simulink model "cn_i_128w_2k_do_al_r302"  (Simulink 6.2)
settings: Solver=ode45  StartTime=0.0  StopTime=1000  RelTol=1e-3
libraries: xbsIndex_r3 x481, xps_library x27, ddc_library x4, reorder_library x3, fft_library x2, pfb_library x2, simulink x1, adcscope_lib x1, delay_lib x1
(part 2 of 4)

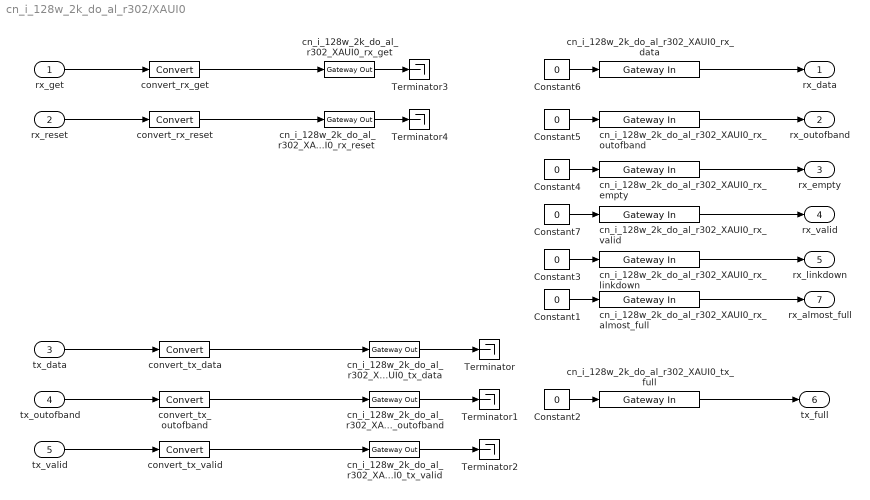
== system cn_i_128w_2k_do_al_r302/XAUI0 ==
  rx_get : Inport  Port=1  LatchInput=off
  rx_reset : Inport  Port=2  LatchInput=off
  tx_data : Inport  Port=3  LatchInput=off
  tx_outofband : Inport  Port=4  LatchInput=off
  tx_valid : Inport  Port=5  LatchInput=off
  Constant{1..7} (7 alike) : Constant  Value=0
  Terminator{,1..4} (5 alike) : Terminator
  cn_i_128w_2k_do_al_r302_XAUI0_rx_almost_full : xbsIndex_r3/Gateway In  arith_type=Boolean  n_bits=1  bin_pt=0  quantization=Truncate  overflow=Wrap  period=1  timing_constraint=None  locs_specified=off  LOCs={}  needs_fixed_name=off  dbl_ovrd=off  show_param=off
      settings: xl_area=[0, 0, 0, 0, 0, 0, 0]
  cn_i_128w_2k_do_al_r302_XAUI0_rx_data : xbsIndex_r3/Gateway In  arith_type=Unsigned  n_bits=64  bin_pt=0  quantization=Truncate  overflow=Wrap  period=1  timing_constraint=None  locs_specified=off  LOCs={}  needs_fixed_name=off  dbl_ovrd=off  show_param=off
      settings: xl_area=[0, 0, 0, 0, 0, 0, 0]
  cn_i_128w_2k_do_al_r302_XAUI0_rx_empty : xbsIndex_r3/Gateway In  arith_type=Boolean  n_bits=1  bin_pt=0  quantization=Truncate  overflow=Wrap  period=1  timing_constraint=None  locs_specified=off  LOCs={}  needs_fixed_name=off  dbl_ovrd=off  show_param=off
      settings: xl_area=[0, 0, 0, 0, 0, 0, 0]
  cn_i_128w_2k_do_al_r302_XAUI0_rx_get : xbsIndex_r3/Gateway Out  output_type=Double  nbits=8  bin_pt=6  arith_type=Boolean  quantization=Truncate  overflow=Wrap  hdl_port=on  timing_constraint=None  locs_specified=off  LOCs={}  needs_fixed_name=off  show_param=off
      settings: xl_area=[0, 0, 0, 0, 0, 0, 0]
  cn_i_128w_2k_do_al_r302_XAUI0_rx_linkdown : xbsIndex_r3/Gateway In  arith_type=Boolean  n_bits=1  bin_pt=0  quantization=Truncate  overflow=Wrap  period=1  timing_constraint=None  locs_specified=off  LOCs={}  needs_fixed_name=off  dbl_ovrd=off  show_param=off
      settings: xl_area=[0, 0, 0, 0, 0, 0, 0]
  cn_i_128w_2k_do_al_r302_XAUI0_rx_outofband : xbsIndex_r3/Gateway In  arith_type=Unsigned  n_bits=8  bin_pt=0  quantization=Truncate  overflow=Wrap  period=1  timing_constraint=None  locs_specified=off  LOCs={}  needs_fixed_name=off  dbl_ovrd=off  show_param=off
      settings: xl_area=[0, 0, 0, 0, 0, 0, 0]
  cn_i_128w_2k_do_al_r302_XAUI0_rx_reset : xbsIndex_r3/Gateway Out  output_type=Double  nbits=8  bin_pt=6  arith_type=Boolean  quantization=Truncate  overflow=Wrap  hdl_port=on  timing_constraint=None  locs_specified=off  LOCs={}  needs_fixed_name=off  show_param=off
      settings: xl_area=[0, 0, 0, 0, 0, 0, 0]
  cn_i_128w_2k_do_al_r302_XAUI0_rx_valid : xbsIndex_r3/Gateway In  arith_type=Boolean  n_bits=1  bin_pt=0  quantization=Truncate  overflow=Wrap  period=1  timing_constraint=None  locs_specified=off  LOCs={}  needs_fixed_name=off  dbl_ovrd=off  show_param=off
      settings: xl_area=[0, 0, 0, 0, 0, 0, 0]
  cn_i_128w_2k_do_al_r302_XAUI0_tx_data : xbsIndex_r3/Gateway Out  output_type=Double  nbits=8  bin_pt=6  arith_type=Boolean  quantization=Truncate  overflow=Wrap  hdl_port=on  timing_constraint=None  locs_specified=off  LOCs={}  needs_fixed_name=off  show_param=off
      settings: xl_area=[0, 0, 0, 0, 0, 0, 0]
  cn_i_128w_2k_do_al_r302_XAUI0_tx_full : xbsIndex_r3/Gateway In  arith_type=Boolean  n_bits=1  bin_pt=0  quantization=Truncate  overflow=Wrap  period=1  timing_constraint=None  locs_specified=off  LOCs={}  needs_fixed_name=off  dbl_ovrd=off  show_param=off
      settings: xl_area=[0, 0, 0, 0, 0, 0, 0]
  cn_i_128w_2k_do_al_r302_XAUI0_tx_outofband : xbsIndex_r3/Gateway Out  output_type=Double  nbits=8  bin_pt=6  arith_type=Boolean  quantization=Truncate  overflow=Wrap  hdl_port=on  timing_constraint=None  locs_specified=off  LOCs={}  needs_fixed_name=off  show_param=off
      settings: xl_area=[0, 0, 0, 0, 0, 0, 0]
  cn_i_128w_2k_do_al_r302_XAUI0_tx_valid : xbsIndex_r3/Gateway Out  output_type=Double  nbits=8  bin_pt=6  arith_type=Boolean  quantization=Truncate  overflow=Wrap  hdl_port=on  timing_constraint=None  locs_specified=off  LOCs={}  needs_fixed_name=off  show_param=off
      settings: xl_area=[0, 0, 0, 0, 0, 0, 0]
  convert_rx_get : xbsIndex_r3/Convert  arith_type=Boolean  n_bits=64  bin_pt=0  quantization=Truncate  overflow=Wrap  latency=0  explicit_period=off  period=1  dbl_ovrd=off  show_param=off  inserted_by_tool=off  pipeline=off
      settings: xl_area=[0, 0, 0, 0, 0, 0, 0]
  convert_rx_reset : xbsIndex_r3/Convert  arith_type=Boolean  n_bits=1  bin_pt=0  quantization=Truncate  overflow=Wrap  latency=0  explicit_period=off  period=1  dbl_ovrd=off  show_param=off  inserted_by_tool=off  pipeline=off
      settings: xl_area=[0, 0, 0, 0, 0, 0, 0]
  convert_tx_data : xbsIndex_r3/Convert  arith_type=Unsigned  n_bits=64  bin_pt=0  quantization=Truncate  overflow=Wrap  latency=0  explicit_period=off  period=1  dbl_ovrd=off  show_param=off  inserted_by_tool=off  pipeline=off
      settings: xl_area=[0, 0, 0, 0, 0, 0, 0]
  convert_tx_outofband : xbsIndex_r3/Convert  arith_type=Unsigned  n_bits=8  bin_pt=0  quantization=Truncate  overflow=Wrap  latency=0  explicit_period=off  period=1  dbl_ovrd=off  show_param=off  inserted_by_tool=off  pipeline=off
      settings: xl_area=[0, 0, 0, 0, 0, 0, 0]
  convert_tx_valid : xbsIndex_r3/Convert  arith_type=Boolean  n_bits=1  bin_pt=0  quantization=Truncate  overflow=Wrap  latency=0  explicit_period=off  period=1  dbl_ovrd=off  show_param=off  inserted_by_tool=off  pipeline=off
      settings: xl_area=[0, 0, 0, 0, 0, 0, 0]
  rx_data : Outport
  rx_outofband : Outport  Port=2
  rx_empty : Outport  Port=3
  rx_valid : Outport  Port=4
  rx_linkdown : Outport  Port=5
  tx_full : Outport  Port=6
  rx_almost_full : Outport  Port=7
  wires:
  Constant1/1 -> cn_i_128w_2k_do_al_r302_XAUI0_rx_almost_full/1
  cn_i_128w_2k_do_al_r302_XAUI0_rx_almost_full/1 -> rx_almost_full/1
  cn_i_128w_2k_do_al_r302_XAUI0_rx_valid/1 -> rx_valid/1
  Constant7/1 -> cn_i_128w_2k_do_al_r302_XAUI0_rx_valid/1
  cn_i_128w_2k_do_al_r302_XAUI0_rx_reset/1 -> Terminator4/1
  cn_i_128w_2k_do_al_r302_XAUI0_rx_get/1 -> Terminator3/1
  Constant6/1 -> cn_i_128w_2k_do_al_r302_XAUI0_rx_data/1
  Constant5/1 -> cn_i_128w_2k_do_al_r302_XAUI0_rx_outofband/1
  Constant4/1 -> cn_i_128w_2k_do_al_r302_XAUI0_rx_empty/1
  Constant3/1 -> cn_i_128w_2k_do_al_r302_XAUI0_rx_linkdown/1
  Constant2/1 -> cn_i_128w_2k_do_al_r302_XAUI0_tx_full/1
  cn_i_128w_2k_do_al_r302_XAUI0_tx_valid/1 -> Terminator2/1
  cn_i_128w_2k_do_al_r302_XAUI0_tx_outofband/1 -> Terminator1/1
  cn_i_128w_2k_do_al_r302_XAUI0_tx_data/1 -> Terminator/1
  cn_i_128w_2k_do_al_r302_XAUI0_tx_full/1 -> tx_full/1
  convert_tx_valid/1 -> cn_i_128w_2k_do_al_r302_XAUI0_tx_valid/1
  tx_valid/1 -> convert_tx_valid/1
  convert_tx_outofband/1 -> cn_i_128w_2k_do_al_r302_XAUI0_tx_outofband/1
  tx_outofband/1 -> convert_tx_outofband/1
  convert_tx_data/1 -> cn_i_128w_2k_do_al_r302_XAUI0_tx_data/1
  tx_data/1 -> convert_tx_data/1
  cn_i_128w_2k_do_al_r302_XAUI0_rx_linkdown/1 -> rx_linkdown/1
  cn_i_128w_2k_do_al_r302_XAUI0_rx_empty/1 -> rx_empty/1
  cn_i_128w_2k_do_al_r302_XAUI0_rx_outofband/1 -> rx_outofband/1
  cn_i_128w_2k_do_al_r302_XAUI0_rx_data/1 -> rx_data/1
  convert_rx_reset/1 -> cn_i_128w_2k_do_al_r302_XAUI0_rx_reset/1
  rx_reset/1 -> convert_rx_reset/1
  convert_rx_get/1 -> cn_i_128w_2k_do_al_r302_XAUI0_rx_get/1
  rx_get/1 -> convert_rx_get/1

== system cn_i_128w_2k_do_al_r302/calc_adc_sum_sq1 ==
  pol_in : Inport  Port=1  LatchInput=off
  accum_rst : Inport  Port=2  LatchInput=off
  Accumulator : xbsIndex_r3/Accumulator  n_bits=32  overflow=Wrap  operation=Add  scale=1  explicit_period=off  period=1  rst=on  hasbypass=off  en=off  dbl_ovrd=off  show_param=off  gen_core=off  use_rpm=on
      settings: xl_area=[0, 0, 0, 0, 0, 0, 0]
  Counter : xbsIndex_r3/Counter  cnt_type=Free Running  n_bits=2  bin_pt=0  arith_type=Unsigned  start_count=0  cnt_to=Inf  cnt_by_val=1  operation=Up  explicit_period=off  period=1  load_pin=off  rst=off  en=off  dbl_ovrd=off  show_param=off  use_rpm=on  gen_core=off
      settings: xl_area=[0, 0, 0, 0, 0, 0, 0]
  Mult : xbsIndex_r3/Mult  precision=Full  arith_type="Signed  (2's comp)"  n_bits=8  bin_pt=2  quantization=Truncate  overflow=Wrap  latency=2  explicit_period=on  period=1  en=off  dbl_ovrd=off  show_param=off  mult_type=Parallel  oversample=2  use_embedded=off  pipeline=on  use_rpm=on  placement_style=Rectangular Shape  gen_core=off
      settings: xl_area=[0, 0, 0, 0, 0, 0, 0]
  Mux : xbsIndex_r3/Mux  inputs=4  precision=Full  arith_type="Signed  (2's comp)"  n_bits=8  bin_pt=2  quantization=Truncate  overflow=Wrap  latency=1  explicit_period=off  period=1  en=off  dbl_ovrd=off  show_param=off  mux_type=off  use_rpm=off  gen_core=off
      settings: xl_area=[0, 0, 0, 0, 0, 0, 0]
  Register : xbsIndex_r3/Register  init=0  reg_only_valid=off  explicit_period=off  period=1  rst=off  en=on  out_en=off  dbl_ovrd=off  show_param=off
      settings: xl_area=[0, 0, 0, 0, 0, 0, 0]
  decat4 : Subsystem
  sum_sq : Outport
  wires:
  Mult/1 -> Accumulator/1
  Accumulator/1 -> Register/1
  Register/1 -> sum_sq/1
  Mux/1 -> Mult/1, Mult/2
  Counter/1 -> Mux/1
  accum_rst/1 -> Accumulator/2, Register/2
  pol_in/1 -> decat4/1(In1)
  decat4/1(Out1) -> Mux/2
  decat4/2(Out2) -> Mux/4
  decat4/3(Out3) -> Mux/3
  decat4/4(Out4) -> Mux/5

== system cn_i_128w_2k_do_al_r302/calc_adc_sum_sq2 ==
  pol_in : Inport  Port=1  LatchInput=off
  accum_rst : Inport  Port=2  LatchInput=off
  Accumulator : xbsIndex_r3/Accumulator  n_bits=32  overflow=Wrap  operation=Add  scale=1  explicit_period=off  period=1  rst=on  hasbypass=off  en=off  dbl_ovrd=off  show_param=off  gen_core=off  use_rpm=on
      settings: xl_area=[0, 0, 0, 0, 0, 0, 0]
  Counter : xbsIndex_r3/Counter  cnt_type=Free Running  n_bits=2  bin_pt=0  arith_type=Unsigned  start_count=0  cnt_to=Inf  cnt_by_val=1  operation=Up  explicit_period=off  period=1  load_pin=off  rst=off  en=off  dbl_ovrd=off  show_param=off  use_rpm=on  gen_core=off
      settings: xl_area=[0, 0, 0, 0, 0, 0, 0]
  Mult : xbsIndex_r3/Mult  precision=Full  arith_type="Signed  (2's comp)"  n_bits=8  bin_pt=2  quantization=Truncate  overflow=Wrap  latency=2  explicit_period=on  period=1  en=off  dbl_ovrd=off  show_param=off  mult_type=Parallel  oversample=2  use_embedded=off  pipeline=on  use_rpm=on  placement_style=Rectangular Shape  gen_core=off
      settings: xl_area=[0, 0, 0, 0, 0, 0, 0]
  Mux : xbsIndex_r3/Mux  inputs=4  precision=Full  arith_type="Signed  (2's comp)"  n_bits=8  bin_pt=2  quantization=Truncate  overflow=Wrap  latency=1  explicit_period=off  period=1  en=off  dbl_ovrd=off  show_param=off  mux_type=off  use_rpm=off  gen_core=off
      settings: xl_area=[0, 0, 0, 0, 0, 0, 0]
  Register : xbsIndex_r3/Register  init=0  reg_only_valid=off  explicit_period=off  period=1  rst=off  en=on  out_en=off  dbl_ovrd=off  show_param=off
      settings: xl_area=[0, 0, 0, 0, 0, 0, 0]
  decat4 : Subsystem
  sum_sq : Outport
  wires:
  Mult/1 -> Accumulator/1
  Accumulator/1 -> Register/1
  Register/1 -> sum_sq/1
  Mux/1 -> Mult/1, Mult/2
  Counter/1 -> Mux/1
  accum_rst/1 -> Accumulator/2, Register/2
  pol_in/1 -> decat4/1(In1)
  decat4/1(Out1) -> Mux/2
  decat4/2(Out2) -> Mux/4
  decat4/3(Out3) -> Mux/3
  decat4/4(Out4) -> Mux/5

== system cn_i_128w_2k_do_al_r302/calc_adc_sum_sq3 ==
  pol_in : Inport  Port=1  LatchInput=off
  accum_rst : Inport  Port=2  LatchInput=off
  Accumulator : xbsIndex_r3/Accumulator  n_bits=32  overflow=Wrap  operation=Add  scale=1  explicit_period=off  period=1  rst=on  hasbypass=off  en=off  dbl_ovrd=off  show_param=off  gen_core=off  use_rpm=on
      settings: xl_area=[0, 0, 0, 0, 0, 0, 0]
  Counter : xbsIndex_r3/Counter  cnt_type=Free Running  n_bits=2  bin_pt=0  arith_type=Unsigned  start_count=0  cnt_to=Inf  cnt_by_val=1  operation=Up  explicit_period=off  period=1  load_pin=off  rst=off  en=off  dbl_ovrd=off  show_param=off  use_rpm=on  gen_core=off
      settings: xl_area=[0, 0, 0, 0, 0, 0, 0]
  Mult : xbsIndex_r3/Mult  precision=Full  arith_type="Signed  (2's comp)"  n_bits=8  bin_pt=2  quantization=Truncate  overflow=Wrap  latency=2  explicit_period=on  period=1  en=off  dbl_ovrd=off  show_param=off  mult_type=Parallel  oversample=2  use_embedded=off  pipeline=on  use_rpm=on  placement_style=Rectangular Shape  gen_core=off
      settings: xl_area=[0, 0, 0, 0, 0, 0, 0]
  Mux : xbsIndex_r3/Mux  inputs=4  precision=Full  arith_type="Signed  (2's comp)"  n_bits=8  bin_pt=2  quantization=Truncate  overflow=Wrap  latency=1  explicit_period=off  period=1  en=off  dbl_ovrd=off  show_param=off  mux_type=off  use_rpm=off  gen_core=off
      settings: xl_area=[0, 0, 0, 0, 0, 0, 0]
  Register : xbsIndex_r3/Register  init=0  reg_only_valid=off  explicit_period=off  period=1  rst=off  en=on  out_en=off  dbl_ovrd=off  show_param=off
      settings: xl_area=[0, 0, 0, 0, 0, 0, 0]
  decat4 : Subsystem
  sum_sq : Outport
  wires:
  Mult/1 -> Accumulator/1
  Accumulator/1 -> Register/1
  Register/1 -> sum_sq/1
  Mux/1 -> Mult/1, Mult/2
  Counter/1 -> Mux/1
  accum_rst/1 -> Accumulator/2, Register/2
  pol_in/1 -> decat4/1(In1)
  decat4/1(Out1) -> Mux/2
  decat4/2(Out2) -> Mux/4
  decat4/3(Out3) -> Mux/3
  decat4/4(Out4) -> Mux/5

== system cn_i_128w_2k_do_al_r302/calc_adc_sum_sq4 ==
  pol_in : Inport  Port=1  LatchInput=off
  accum_rst : Inport  Port=2  LatchInput=off
  Accumulator : xbsIndex_r3/Accumulator  n_bits=32  overflow=Wrap  operation=Add  scale=1  explicit_period=off  period=1  rst=on  hasbypass=off  en=off  dbl_ovrd=off  show_param=off  gen_core=off  use_rpm=on
      settings: xl_area=[0, 0, 0, 0, 0, 0, 0]
  Counter : xbsIndex_r3/Counter  cnt_type=Free Running  n_bits=2  bin_pt=0  arith_type=Unsigned  start_count=0  cnt_to=Inf  cnt_by_val=1  operation=Up  explicit_period=off  period=1  load_pin=off  rst=off  en=off  dbl_ovrd=off  show_param=off  use_rpm=on  gen_core=off
      settings: xl_area=[0, 0, 0, 0, 0, 0, 0]
  Mult : xbsIndex_r3/Mult  precision=Full  arith_type="Signed  (2's comp)"  n_bits=8  bin_pt=2  quantization=Truncate  overflow=Wrap  latency=2  explicit_period=on  period=1  en=off  dbl_ovrd=off  show_param=off  mult_type=Parallel  oversample=2  use_embedded=off  pipeline=on  use_rpm=on  placement_style=Rectangular Shape  gen_core=off
      settings: xl_area=[0, 0, 0, 0, 0, 0, 0]
  Mux : xbsIndex_r3/Mux  inputs=4  precision=Full  arith_type="Signed  (2's comp)"  n_bits=8  bin_pt=2  quantization=Truncate  overflow=Wrap  latency=1  explicit_period=off  period=1  en=off  dbl_ovrd=off  show_param=off  mux_type=off  use_rpm=off  gen_core=off
      settings: xl_area=[0, 0, 0, 0, 0, 0, 0]
  Register : xbsIndex_r3/Register  init=0  reg_only_valid=off  explicit_period=off  period=1  rst=off  en=on  out_en=off  dbl_ovrd=off  show_param=off
      settings: xl_area=[0, 0, 0, 0, 0, 0, 0]
  decat4 : Subsystem
  sum_sq : Outport
  wires:
  Mult/1 -> Accumulator/1
  Accumulator/1 -> Register/1
  Register/1 -> sum_sq/1
  Mux/1 -> Mult/1, Mult/2
  Counter/1 -> Mux/1
  accum_rst/1 -> Accumulator/2, Register/2
  pol_in/1 -> decat4/1(In1)
  decat4/1(Out1) -> Mux/2
  decat4/2(Out2) -> Mux/4
  decat4/3(Out3) -> Mux/3
  decat4/4(Out4) -> Mux/5

== system cn_i_128w_2k_do_al_r302/concat ==
  In1 : Inport  Port=1  LatchInput=off
  In2 : Inport  Port=2  LatchInput=off
  In3 : Inport  Port=3  LatchInput=off
  In4 : Inport  Port=4  LatchInput=off
  Concat2 : xbsIndex_r3/Concat  num_inputs=4  explicit_period=off  period=1  dbl_ovrd=off
  R1 : xbsIndex_r3/Reinterpret  force_arith_type=on  arith_type=Unsigned  force_bin_pt=on  bin_pt=0  force_valid=on
  R2 : xbsIndex_r3/Reinterpret  force_arith_type=on  arith_type=Unsigned  force_bin_pt=on  bin_pt=0  force_valid=on
  R3 : xbsIndex_r3/Reinterpret  force_arith_type=on  arith_type=Unsigned  force_bin_pt=on  bin_pt=0  force_valid=on
  Reinterpret2 : xbsIndex_r3/Reinterpret  force_arith_type=on  arith_type=Unsigned  force_bin_pt=on  bin_pt=0  force_valid=on
  Out1 : Outport
  wires:
  Reinterpret2/1 -> Concat2/1
  R1/1 -> Concat2/2
  R2/1 -> Concat2/3
  R3/1 -> Concat2/4
  In1/1 -> Reinterpret2/1
  In2/1 -> R1/1
  In3/1 -> R2/1
  In4/1 -> R3/1
  Concat2/1 -> Out1/1

== system cn_i_128w_2k_do_al_r302/concat4 ==
  In1 : Inport  Port=1  LatchInput=off
  In2 : Inport  Port=2  LatchInput=off
  In3 : Inport  Port=3  LatchInput=off
  In4 : Inport  Port=4  LatchInput=off
  Concat2 : xbsIndex_r3/Concat  num_inputs=4  explicit_period=off  period=1  dbl_ovrd=off
  R1 : xbsIndex_r3/Reinterpret  force_arith_type=on  arith_type=Unsigned  force_bin_pt=on  bin_pt=0  force_valid=on
  R2 : xbsIndex_r3/Reinterpret  force_arith_type=on  arith_type=Unsigned  force_bin_pt=on  bin_pt=0  force_valid=on
  R3 : xbsIndex_r3/Reinterpret  force_arith_type=on  arith_type=Unsigned  force_bin_pt=on  bin_pt=0  force_valid=on
  Reinterpret2 : xbsIndex_r3/Reinterpret  force_arith_type=on  arith_type=Unsigned  force_bin_pt=on  bin_pt=0  force_valid=on
  Out1 : Outport
  wires:
  Concat2/1 -> Out1/1
  In4/1 -> R3/1
  In3/1 -> R2/1
  In2/1 -> R1/1
  In1/1 -> Reinterpret2/1
  R3/1 -> Concat2/4
  R2/1 -> Concat2/3
  R1/1 -> Concat2/2
  Reinterpret2/1 -> Concat2/1

== system cn_i_128w_2k_do_al_r302/concat5 ==
  In1 : Inport  Port=1  LatchInput=off
  In2 : Inport  Port=2  LatchInput=off
  In3 : Inport  Port=3  LatchInput=off
  In4 : Inport  Port=4  LatchInput=off
  Concat2 : xbsIndex_r3/Concat  num_inputs=4  explicit_period=off  period=1  dbl_ovrd=off
  R1 : xbsIndex_r3/Reinterpret  force_arith_type=on  arith_type=Unsigned  force_bin_pt=on  bin_pt=0  force_valid=on
  R2 : xbsIndex_r3/Reinterpret  force_arith_type=on  arith_type=Unsigned  force_bin_pt=on  bin_pt=0  force_valid=on
  R3 : xbsIndex_r3/Reinterpret  force_arith_type=on  arith_type=Unsigned  force_bin_pt=on  bin_pt=0  force_valid=on
  Reinterpret2 : xbsIndex_r3/Reinterpret  force_arith_type=on  arith_type=Unsigned  force_bin_pt=on  bin_pt=0  force_valid=on
  Out1 : Outport
  wires:
  Reinterpret2/1 -> Concat2/1
  R1/1 -> Concat2/2
  R2/1 -> Concat2/3
  R3/1 -> Concat2/4
  In1/1 -> Reinterpret2/1
  In2/1 -> R1/1
  In3/1 -> R2/1
  In4/1 -> R3/1
  Concat2/1 -> Out1/1

== system cn_i_128w_2k_do_al_r302/concat6 ==
  In1 : Inport  Port=1  LatchInput=off
  In2 : Inport  Port=2  LatchInput=off
  In3 : Inport  Port=3  LatchInput=off
  In4 : Inport  Port=4  LatchInput=off
  Concat2 : xbsIndex_r3/Concat  num_inputs=4  explicit_period=off  period=1  dbl_ovrd=off
  R1 : xbsIndex_r3/Reinterpret  force_arith_type=on  arith_type=Unsigned  force_bin_pt=on  bin_pt=0  force_valid=on
  R2 : xbsIndex_r3/Reinterpret  force_arith_type=on  arith_type=Unsigned  force_bin_pt=on  bin_pt=0  force_valid=on
  R3 : xbsIndex_r3/Reinterpret  force_arith_type=on  arith_type=Unsigned  force_bin_pt=on  bin_pt=0  force_valid=on
  Reinterpret2 : xbsIndex_r3/Reinterpret  force_arith_type=on  arith_type=Unsigned  force_bin_pt=on  bin_pt=0  force_valid=on
  Out1 : Outport
  wires:
  Concat2/1 -> Out1/1
  In4/1 -> R3/1
  In3/1 -> R2/1
  In2/1 -> R1/1
  In1/1 -> Reinterpret2/1
  R3/1 -> Concat2/4
  R2/1 -> Concat2/3
  R1/1 -> Concat2/2
  Reinterpret2/1 -> Concat2/1

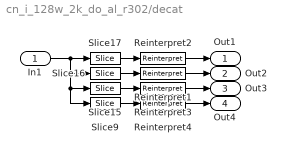
== system cn_i_128w_2k_do_al_r302/decat ==
  In1 : Inport  Port=1  LatchInput=off
  Reinterpret{1..4} (4 alike) : xbsIndex_r3/Reinterpret  force_arith_type=on  arith_type="Signed  (2's comp)"  force_bin_pt=on  bin_pt=7  force_valid=on
  Slice15 : xbsIndex_r3/Slice  mode=Lower Bit Location + Width  nbits=8  bit1=0  base1=MSB of Input  bit0=8  base0=LSB of Input  boolean_output=off  explicit_period=off  period=1  dbl_ovrd=off
  Slice16 : xbsIndex_r3/Slice  mode=Lower Bit Location + Width  nbits=8  bit1=0  base1=MSB of Input  bit0=16  base0=LSB of Input  boolean_output=off  explicit_period=off  period=1  dbl_ovrd=off
  Slice17 : xbsIndex_r3/Slice  mode=Lower Bit Location + Width  nbits=8  bit1=0  base1=MSB of Input  bit0=24  base0=LSB of Input  boolean_output=off  explicit_period=off  period=1  dbl_ovrd=off
  Slice9 : xbsIndex_r3/Slice  mode=Lower Bit Location + Width  nbits=8  bit1=0  base1=MSB of Input  bit0=0  base0=LSB of Input  boolean_output=off  explicit_period=off  period=1  dbl_ovrd=off
  Out1 : Outport
  Out2 : Outport  Port=2
  Out3 : Outport  Port=3
  Out4 : Outport  Port=4
  wires:
  In1/1 -> Slice17/1, Slice16/1, Slice9/1, Slice15/1
  Slice17/1 -> Reinterpret2/1
  Slice16/1 -> Reinterpret1/1
  Slice15/1 -> Reinterpret3/1
  Slice9/1 -> Reinterpret4/1
  Reinterpret2/1 -> Out1/1
  Reinterpret1/1 -> Out2/1
  Reinterpret3/1 -> Out3/1
  Reinterpret4/1 -> Out4/1

== system cn_i_128w_2k_do_al_r302/decat1 ==
  In1 : Inport  Port=1  LatchInput=off
  Reinterpret{1..4} (4 alike) : xbsIndex_r3/Reinterpret  force_arith_type=on  arith_type="Signed  (2's comp)"  force_bin_pt=on  bin_pt=7  force_valid=on
  Slice15 : xbsIndex_r3/Slice  mode=Lower Bit Location + Width  nbits=8  bit1=0  base1=MSB of Input  bit0=8  base0=LSB of Input  boolean_output=off  explicit_period=off  period=1  dbl_ovrd=off
  Slice16 : xbsIndex_r3/Slice  mode=Lower Bit Location + Width  nbits=8  bit1=0  base1=MSB of Input  bit0=16  base0=LSB of Input  boolean_output=off  explicit_period=off  period=1  dbl_ovrd=off
  Slice17 : xbsIndex_r3/Slice  mode=Lower Bit Location + Width  nbits=8  bit1=0  base1=MSB of Input  bit0=24  base0=LSB of Input  boolean_output=off  explicit_period=off  period=1  dbl_ovrd=off
  Slice9 : xbsIndex_r3/Slice  mode=Lower Bit Location + Width  nbits=8  bit1=0  base1=MSB of Input  bit0=0  base0=LSB of Input  boolean_output=off  explicit_period=off  period=1  dbl_ovrd=off
  Out1 : Outport
  Out2 : Outport  Port=2
  Out3 : Outport  Port=3
  Out4 : Outport  Port=4
  wires:
  Reinterpret4/1 -> Out4/1
  Reinterpret3/1 -> Out3/1
  Reinterpret1/1 -> Out2/1
  Reinterpret2/1 -> Out1/1
  Slice9/1 -> Reinterpret4/1
  Slice15/1 -> Reinterpret3/1
  Slice16/1 -> Reinterpret1/1
  Slice17/1 -> Reinterpret2/1
  In1/1 -> Slice15/1, Slice9/1, Slice16/1, Slice17/1

== system cn_i_128w_2k_do_al_r302/decat2 ==
  In1 : Inport  Port=1  LatchInput=off
  Reinterpret{1..4} (4 alike) : xbsIndex_r3/Reinterpret  force_arith_type=on  arith_type="Signed  (2's comp)"  force_bin_pt=on  bin_pt=7  force_valid=on
  Slice15 : xbsIndex_r3/Slice  mode=Lower Bit Location + Width  nbits=8  bit1=0  base1=MSB of Input  bit0=8  base0=LSB of Input  boolean_output=off  explicit_period=off  period=1  dbl_ovrd=off
  Slice16 : xbsIndex_r3/Slice  mode=Lower Bit Location + Width  nbits=8  bit1=0  base1=MSB of Input  bit0=16  base0=LSB of Input  boolean_output=off  explicit_period=off  period=1  dbl_ovrd=off
  Slice17 : xbsIndex_r3/Slice  mode=Lower Bit Location + Width  nbits=8  bit1=0  base1=MSB of Input  bit0=24  base0=LSB of Input  boolean_output=off  explicit_period=off  period=1  dbl_ovrd=off
  Slice9 : xbsIndex_r3/Slice  mode=Lower Bit Location + Width  nbits=8  bit1=0  base1=MSB of Input  bit0=0  base0=LSB of Input  boolean_output=off  explicit_period=off  period=1  dbl_ovrd=off
  Out1 : Outport
  Out2 : Outport  Port=2
  Out3 : Outport  Port=3
  Out4 : Outport  Port=4
  wires:
  Reinterpret4/1 -> Out4/1
  Reinterpret3/1 -> Out3/1
  Reinterpret1/1 -> Out2/1
  Reinterpret2/1 -> Out1/1
  Slice9/1 -> Reinterpret4/1
  Slice15/1 -> Reinterpret3/1
  Slice16/1 -> Reinterpret1/1
  Slice17/1 -> Reinterpret2/1
  In1/1 -> Slice15/1, Slice9/1, Slice16/1, Slice17/1

== system cn_i_128w_2k_do_al_r302/decat3 ==
  In1 : Inport  Port=1  LatchInput=off
  Reinterpret{1..4} (4 alike) : xbsIndex_r3/Reinterpret  force_arith_type=on  arith_type="Signed  (2's comp)"  force_bin_pt=on  bin_pt=7  force_valid=on
  Slice15 : xbsIndex_r3/Slice  mode=Lower Bit Location + Width  nbits=8  bit1=0  base1=MSB of Input  bit0=8  base0=LSB of Input  boolean_output=off  explicit_period=off  period=1  dbl_ovrd=off
  Slice16 : xbsIndex_r3/Slice  mode=Lower Bit Location + Width  nbits=8  bit1=0  base1=MSB of Input  bit0=16  base0=LSB of Input  boolean_output=off  explicit_period=off  period=1  dbl_ovrd=off
  Slice17 : xbsIndex_r3/Slice  mode=Lower Bit Location + Width  nbits=8  bit1=0  base1=MSB of Input  bit0=24  base0=LSB of Input  boolean_output=off  explicit_period=off  period=1  dbl_ovrd=off
  Slice9 : xbsIndex_r3/Slice  mode=Lower Bit Location + Width  nbits=8  bit1=0  base1=MSB of Input  bit0=0  base0=LSB of Input  boolean_output=off  explicit_period=off  period=1  dbl_ovrd=off
  Out1 : Outport
  Out2 : Outport  Port=2
  Out3 : Outport  Port=3
  Out4 : Outport  Port=4
  wires:
  In1/1 -> Slice17/1, Slice16/1, Slice9/1, Slice15/1
  Slice17/1 -> Reinterpret2/1
  Slice16/1 -> Reinterpret1/1
  Slice15/1 -> Reinterpret3/1
  Slice9/1 -> Reinterpret4/1
  Reinterpret2/1 -> Out1/1
  Reinterpret1/1 -> Out2/1
  Reinterpret3/1 -> Out3/1
  Reinterpret4/1 -> Out4/1

== system cn_i_128w_2k_do_al_r302/downshift ==
  din : Inport  Port=1  LatchInput=off
  Concat : xbsIndex_r3/Concat  num_inputs=2  explicit_period=off  period=1  dbl_ovrd=off
  Convert1 : xbsIndex_r3/Convert  arith_type="Signed  (2's comp)"  n_bits=18  bin_pt=15  quantization="Round  (unbiased: Even Values)"  overflow=Wrap  latency=2  explicit_period=off  period=1  dbl_ovrd=off  show_param=off  inserted_by_tool=off  pipeline=off
      settings: xl_area=[0, 0, 0, 0, 0, 0, 0]
  Convert2 : xbsIndex_r3/Convert  arith_type="Signed  (2's comp)"  n_bits=18  bin_pt=15  quantization="Round  (unbiased: Even Values)"  overflow=Wrap  latency=2  explicit_period=off  period=1  dbl_ovrd=off  show_param=off  inserted_by_tool=off  pipeline=off
      settings: xl_area=[0, 0, 0, 0, 0, 0, 0]
  Reinterpret : xbsIndex_r3/Reinterpret  force_arith_type=on  arith_type="Signed  (2's comp)"  force_bin_pt=on  bin_pt=17  force_valid=on
  Reinterpret1 : xbsIndex_r3/Reinterpret  force_arith_type=on  arith_type="Signed  (2's comp)"  force_bin_pt=on  bin_pt=17  force_valid=on
  Reinterpret3 : xbsIndex_r3/Reinterpret  force_arith_type=on  arith_type=Unsigned  force_bin_pt=on  bin_pt=0  force_valid=on
  Reinterpret4 : xbsIndex_r3/Reinterpret  force_arith_type=on  arith_type=Unsigned  force_bin_pt=on  bin_pt=0  force_valid=on
  Slice2 : xbsIndex_r3/Slice  mode=Upper Bit Location + Width  nbits=18  bit1=0  base1=MSB of Input  bit0=0  base0=LSB of Input  boolean_output=off  explicit_period=off  period=1  dbl_ovrd=off
  Slice20 : xbsIndex_r3/Slice  mode=Lower Bit Location + Width  nbits=18  bit1=0  base1=MSB of Input  bit0=0  base0=LSB of Input  boolean_output=off  explicit_period=off  period=1  dbl_ovrd=off
  dout : Outport
  wires:
  Slice2/1 -> Reinterpret/1
  Slice20/1 -> Reinterpret1/1
  din/1 -> Slice2/1, Slice20/1
  Reinterpret3/1 -> Concat/1
  Reinterpret4/1 -> Concat/2
  Concat/1 -> dout/1
  Reinterpret/1 -> Convert2/1
  Reinterpret1/1 -> Convert1/1
  Convert2/1 -> Reinterpret3/1
  Convert1/1 -> Reinterpret4/1

== system cn_i_128w_2k_do_al_r302/downshift1 ==
  din : Inport  Port=1  LatchInput=off
  Concat : xbsIndex_r3/Concat  num_inputs=2  explicit_period=off  period=1  dbl_ovrd=off
  Convert1 : xbsIndex_r3/Convert  arith_type="Signed  (2's comp)"  n_bits=18  bin_pt=15  quantization="Round  (unbiased: Even Values)"  overflow=Wrap  latency=2  explicit_period=off  period=1  dbl_ovrd=off  show_param=off  inserted_by_tool=off  pipeline=off
      settings: xl_area=[0, 0, 0, 0, 0, 0, 0]
  Convert2 : xbsIndex_r3/Convert  arith_type="Signed  (2's comp)"  n_bits=18  bin_pt=15  quantization="Round  (unbiased: Even Values)"  overflow=Wrap  latency=2  explicit_period=off  period=1  dbl_ovrd=off  show_param=off  inserted_by_tool=off  pipeline=off
      settings: xl_area=[0, 0, 0, 0, 0, 0, 0]
  Reinterpret : xbsIndex_r3/Reinterpret  force_arith_type=on  arith_type="Signed  (2's comp)"  force_bin_pt=on  bin_pt=17  force_valid=on
  Reinterpret1 : xbsIndex_r3/Reinterpret  force_arith_type=on  arith_type="Signed  (2's comp)"  force_bin_pt=on  bin_pt=17  force_valid=on
  Reinterpret3 : xbsIndex_r3/Reinterpret  force_arith_type=on  arith_type=Unsigned  force_bin_pt=on  bin_pt=0  force_valid=on
  Reinterpret4 : xbsIndex_r3/Reinterpret  force_arith_type=on  arith_type=Unsigned  force_bin_pt=on  bin_pt=0  force_valid=on
  Slice2 : xbsIndex_r3/Slice  mode=Upper Bit Location + Width  nbits=18  bit1=0  base1=MSB of Input  bit0=0  base0=LSB of Input  boolean_output=off  explicit_period=off  period=1  dbl_ovrd=off
  Slice20 : xbsIndex_r3/Slice  mode=Lower Bit Location + Width  nbits=18  bit1=0  base1=MSB of Input  bit0=0  base0=LSB of Input  boolean_output=off  explicit_period=off  period=1  dbl_ovrd=off
  dout : Outport
  wires:
  Convert1/1 -> Reinterpret4/1
  Convert2/1 -> Reinterpret3/1
  Reinterpret1/1 -> Convert1/1
  Reinterpret/1 -> Convert2/1
  Concat/1 -> dout/1
  Reinterpret4/1 -> Concat/2
  Reinterpret3/1 -> Concat/1
  din/1 -> Slice20/1, Slice2/1
  Slice20/1 -> Reinterpret1/1
  Slice2/1 -> Reinterpret/1

== system cn_i_128w_2k_do_al_r302/downshift2 ==
  din : Inport  Port=1  LatchInput=off
  Concat : xbsIndex_r3/Concat  num_inputs=2  explicit_period=off  period=1  dbl_ovrd=off
  Convert1 : xbsIndex_r3/Convert  arith_type="Signed  (2's comp)"  n_bits=18  bin_pt=15  quantization="Round  (unbiased: Even Values)"  overflow=Wrap  latency=2  explicit_period=off  period=1  dbl_ovrd=off  show_param=off  inserted_by_tool=off  pipeline=off
      settings: xl_area=[0, 0, 0, 0, 0, 0, 0]
  Convert2 : xbsIndex_r3/Convert  arith_type="Signed  (2's comp)"  n_bits=18  bin_pt=15  quantization="Round  (unbiased: Even Values)"  overflow=Wrap  latency=2  explicit_period=off  period=1  dbl_ovrd=off  show_param=off  inserted_by_tool=off  pipeline=off
      settings: xl_area=[0, 0, 0, 0, 0, 0, 0]
  Reinterpret : xbsIndex_r3/Reinterpret  force_arith_type=on  arith_type="Signed  (2's comp)"  force_bin_pt=on  bin_pt=17  force_valid=on
  Reinterpret1 : xbsIndex_r3/Reinterpret  force_arith_type=on  arith_type="Signed  (2's comp)"  force_bin_pt=on  bin_pt=17  force_valid=on
  Reinterpret3 : xbsIndex_r3/Reinterpret  force_arith_type=on  arith_type=Unsigned  force_bin_pt=on  bin_pt=0  force_valid=on
  Reinterpret4 : xbsIndex_r3/Reinterpret  force_arith_type=on  arith_type=Unsigned  force_bin_pt=on  bin_pt=0  force_valid=on
  Slice2 : xbsIndex_r3/Slice  mode=Upper Bit Location + Width  nbits=18  bit1=0  base1=MSB of Input  bit0=0  base0=LSB of Input  boolean_output=off  explicit_period=off  period=1  dbl_ovrd=off
  Slice20 : xbsIndex_r3/Slice  mode=Lower Bit Location + Width  nbits=18  bit1=0  base1=MSB of Input  bit0=0  base0=LSB of Input  boolean_output=off  explicit_period=off  period=1  dbl_ovrd=off
  dout : Outport
  wires:
  Convert1/1 -> Reinterpret4/1
  Convert2/1 -> Reinterpret3/1
  Reinterpret1/1 -> Convert1/1
  Reinterpret/1 -> Convert2/1
  Concat/1 -> dout/1
  Reinterpret4/1 -> Concat/2
  Reinterpret3/1 -> Concat/1
  din/1 -> Slice20/1, Slice2/1
  Slice20/1 -> Reinterpret1/1
  Slice2/1 -> Reinterpret/1

== system cn_i_128w_2k_do_al_r302/downshift3 ==
  din : Inport  Port=1  LatchInput=off
  Concat : xbsIndex_r3/Concat  num_inputs=2  explicit_period=off  period=1  dbl_ovrd=off
  Convert1 : xbsIndex_r3/Convert  arith_type="Signed  (2's comp)"  n_bits=18  bin_pt=15  quantization="Round  (unbiased: Even Values)"  overflow=Wrap  latency=2  explicit_period=off  period=1  dbl_ovrd=off  show_param=off  inserted_by_tool=off  pipeline=off
      settings: xl_area=[0, 0, 0, 0, 0, 0, 0]
  Convert2 : xbsIndex_r3/Convert  arith_type="Signed  (2's comp)"  n_bits=18  bin_pt=15  quantization="Round  (unbiased: Even Values)"  overflow=Wrap  latency=2  explicit_period=off  period=1  dbl_ovrd=off  show_param=off  inserted_by_tool=off  pipeline=off
      settings: xl_area=[0, 0, 0, 0, 0, 0, 0]
  Reinterpret : xbsIndex_r3/Reinterpret  force_arith_type=on  arith_type="Signed  (2's comp)"  force_bin_pt=on  bin_pt=17  force_valid=on
  Reinterpret1 : xbsIndex_r3/Reinterpret  force_arith_type=on  arith_type="Signed  (2's comp)"  force_bin_pt=on  bin_pt=17  force_valid=on
  Reinterpret3 : xbsIndex_r3/Reinterpret  force_arith_type=on  arith_type=Unsigned  force_bin_pt=on  bin_pt=0  force_valid=on
  Reinterpret4 : xbsIndex_r3/Reinterpret  force_arith_type=on  arith_type=Unsigned  force_bin_pt=on  bin_pt=0  force_valid=on
  Slice2 : xbsIndex_r3/Slice  mode=Upper Bit Location + Width  nbits=18  bit1=0  base1=MSB of Input  bit0=0  base0=LSB of Input  boolean_output=off  explicit_period=off  period=1  dbl_ovrd=off
  Slice20 : xbsIndex_r3/Slice  mode=Lower Bit Location + Width  nbits=18  bit1=0  base1=MSB of Input  bit0=0  base0=LSB of Input  boolean_output=off  explicit_period=off  period=1  dbl_ovrd=off
  dout : Outport
  wires:
  Slice2/1 -> Reinterpret/1
  Slice20/1 -> Reinterpret1/1
  din/1 -> Slice2/1, Slice20/1
  Reinterpret3/1 -> Concat/1
  Reinterpret4/1 -> Concat/2
  Concat/1 -> dout/1
  Reinterpret/1 -> Convert2/1
  Reinterpret1/1 -> Convert1/1
  Convert2/1 -> Reinterpret3/1
  Convert1/1 -> Reinterpret4/1

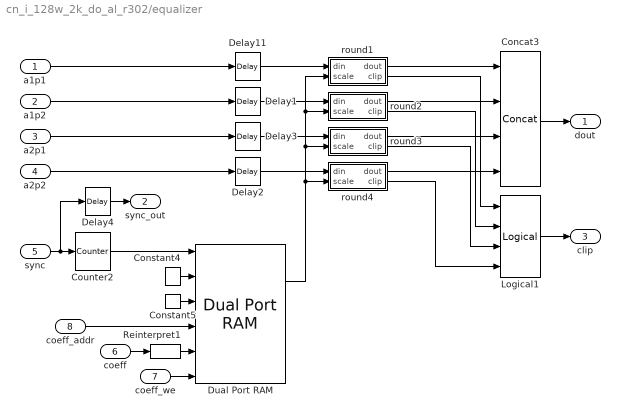
== system cn_i_128w_2k_do_al_r302/equalizer ==
  a1p1 : Inport  Port=1  LatchInput=off
  a1p2 : Inport  Port=2  LatchInput=off
  a2p1 : Inport  Port=3  LatchInput=off
  a2p2 : Inport  Port=4  LatchInput=off
  sync : Inport  Port=5  LatchInput=off
  coeff : Inport  Port=6  LatchInput=off
  coeff_we : Inport  Port=7  LatchInput=off
  coeff_addr : Inport  Port=8  LatchInput=off
  Concat3 : xbsIndex_r3/Concat  num_inputs=4  explicit_period=off  period=1  dbl_ovrd=off
  Constant4 : xbsIndex_r3/Constant  const=0  equ=P=C  arith_type=Unsigned  n_bits=17  bin_pt=3  opselect=C  inp2=PCIN>>17  opr=+  inp1=P  carry=CIN  iostate=0  explicit_period=on  period=1  dbl_ovrd=off
  Constant5 : xbsIndex_r3/Constant  const=0  equ=P=C  arith_type=Boolean  n_bits=1  bin_pt=0  opselect=C  inp2=PCIN>>17  opr=+  inp1=P  carry=CIN  iostate=0  explicit_period=on  period=1  dbl_ovrd=off
  Counter2 : xbsIndex_r3/Counter  cnt_type=Free Running  n_bits=11  bin_pt=0  arith_type=Unsigned  start_count=0  cnt_to=Inf  cnt_by_val=1  operation=Up  explicit_period=off  period=1  load_pin=off  rst=on  en=off  dbl_ovrd=off  show_param=off  use_rpm=on  gen_core=off
      settings: xl_area=[0, 0, 0, 0, 0, 0, 0]
  Delay{1..3,11} (4 alike) : xbsIndex_r3/Delay  latency=1  reg_retiming=off  explicit_period=off  period=1  en=off  accept_only_valid=off  init_zero=on  dbl_ovrd=off  show_param=off
      settings: xl_area=[0, 0, 0, 0, 0, 0, 0]
  Delay4 : xbsIndex_r3/Delay  latency=5  reg_retiming=off  explicit_period=off  period=1  en=off  accept_only_valid=off  init_zero=on  dbl_ovrd=off  show_param=off
      settings: xl_area=[0, 0, 0, 0, 0, 0, 0]
  Dual Port RAM : xbsIndex_r3/Dual Port RAM  depth=2^11  initVector=2^12  write_mode_A=Read After Write  write_mode_B=Read After Write  latency=1  mem_collision=off  init_zero=on  explicit_period=off  period=1  dbl_ovrd=off  rst_a=off  init_a=0  rst_b=off  init_b=0  show_param=off  distributed_mem=off  use_rpm=off  gen_core=off
      settings: xl_area=[0, 0, 0, 0, 0, 0, 0]
  Logical1 : xbsIndex_r3/Logical  logical_function=OR  inputs=4  precision=Full  arith_type=Unsigned  n_bits=8  bin_pt=2  align_bp=on  latency=1  explicit_period=off  period=1  en=off  dbl_ovrd=off  show_param=off
      settings: xl_area=[0, 0, 0, 0, 0, 0, 0]
  Reinterpret1 : xbsIndex_r3/Reinterpret  force_arith_type=on  arith_type=Unsigned  force_bin_pt=on  bin_pt=3  force_valid=on
  round1 : Subsystem
  round2 : Subsystem
  round3 : Subsystem
  round4 : Subsystem
  dout : Outport
  sync_out : Outport  Port=2
  clip : Outport  Port=3
  wires:
  Counter2/1 -> Dual Port RAM/1
  Constant4/1 -> Dual Port RAM/2
  Constant5/1 -> Dual Port RAM/3
  coeff_addr/1 -> Dual Port RAM/4
  coeff_we/1 -> Dual Port RAM/6
  Reinterpret1/1 -> Dual Port RAM/5
  sync/1 -> Counter2/1, Delay4/1
  Dual Port RAM/1 -> round1/2(scale), round2/2(scale), round3/2(scale), round4/2(scale)
  coeff/1 -> Reinterpret1/1
  round1/1(dout) -> Concat3/1
  round2/1(dout) -> Concat3/2
  round3/1(dout) -> Concat3/3
  round4/1(dout) -> Concat3/4
  Delay11/1 -> round1/1(din)
  Delay1/1 -> round2/1(din)
  Delay3/1 -> round3/1(din)
  Delay2/1 -> round4/1(din)
  a1p1/1 -> Delay11/1
  a1p2/1 -> Delay1/1
  a2p1/1 -> Delay3/1
  a2p2/1 -> Delay2/1
  Concat3/1 -> dout/1
  Delay4/1 -> sync_out/1
  round1/2(clip) -> Logical1/1
  round2/2(clip) -> Logical1/2
  round3/2(clip) -> Logical1/3
  round4/2(clip) -> Logical1/4
  Logical1/1 -> clip/1

== system cn_i_128w_2k_do_al_r302/fft_tvg ==
  din : Inport  Port=1  LatchInput=off
  sync : Inport  Port=2  LatchInput=off
  use_tvg : Inport  Port=3  LatchInput=off
  Constant4 : xbsIndex_r3/Constant  const=0  equ=P=C  arith_type=Unsigned  n_bits=32  bin_pt=0  opselect=C  inp2=PCIN>>17  opr=+  inp1=P  carry=CIN  iostate=0  explicit_period=on  period=1  dbl_ovrd=off
  Counter3 : xbsIndex_r3/Counter  cnt_type=Free Running  n_bits=12  bin_pt=0  arith_type=Unsigned  start_count=0  cnt_to=Inf  cnt_by_val=1  operation=Up  explicit_period=off  period=1  load_pin=off  rst=on  en=off  dbl_ovrd=off  show_param=off  use_rpm=on  gen_core=off
      settings: xl_area=[0, 0, 0, 0, 0, 0, 0]
  Inverter : xbsIndex_r3/Inverter  latency=0  explicit_period=off  period=1  en=off  dbl_ovrd=off  show_param=off
      settings: xl_area=[0, 0, 0, 0, 0, 0, 0]
  Logical4 : xbsIndex_r3/Logical  logical_function=XOR  inputs=2  precision=Full  arith_type=Unsigned  n_bits=8  bin_pt=2  align_bp=on  latency=0  explicit_period=off  period=1  en=off  dbl_ovrd=off  show_param=off
      settings: xl_area=[0, 0, 0, 0, 0, 0, 0]
  Mux1 : xbsIndex_r3/Mux  inputs=2  precision=Full  arith_type="Signed  (2's comp)"  n_bits=8  bin_pt=2  quantization=Truncate  overflow=Wrap  latency=0  explicit_period=off  period=1  en=off  dbl_ovrd=off  show_param=off  mux_type=off  use_rpm=off  gen_core=off
      settings: xl_area=[0, 0, 0, 0, 0, 0, 0]
  Mux2 : xbsIndex_r3/Mux  inputs=2  precision=Full  arith_type="Signed  (2's comp)"  n_bits=8  bin_pt=2  quantization=Truncate  overflow=Wrap  latency=0  explicit_period=off  period=1  en=off  dbl_ovrd=off  show_param=off  mux_type=off  use_rpm=off  gen_core=off
      settings: xl_area=[0, 0, 0, 0, 0, 0, 0]
  Slice1 : xbsIndex_r3/Slice  mode=Lower Bit Location + Width  nbits=1  bit1=0  base1=MSB of Input  bit0=0  base0=LSB of Input  boolean_output=off  explicit_period=off  period=1  dbl_ovrd=off
  Slice11 : xbsIndex_r3/Slice  mode=Upper Bit Location + Width  nbits=1  bit1=0  base1=MSB of Input  bit0=0  base0=LSB of Input  boolean_output=off  explicit_period=off  period=1  dbl_ovrd=off
  dout : Outport
  sync_out : Outport  Port=2
  wires:
  use_tvg/1 -> Mux1/1
  din/1 -> Mux1/2
  Mux1/1 -> dout/1
  sync/1 -> Counter3/1, sync_out/1
  Counter3/1 -> Slice1/1, Slice11/1
  Slice11/1 -> Logical4/1
  Slice1/1 -> Logical4/2
  Logical4/1 -> Mux2/1
  Constant4/1 -> Mux2/2, Inverter/1
  Inverter/1 -> Mux2/3
  Mux2/1 -> Mux1/3

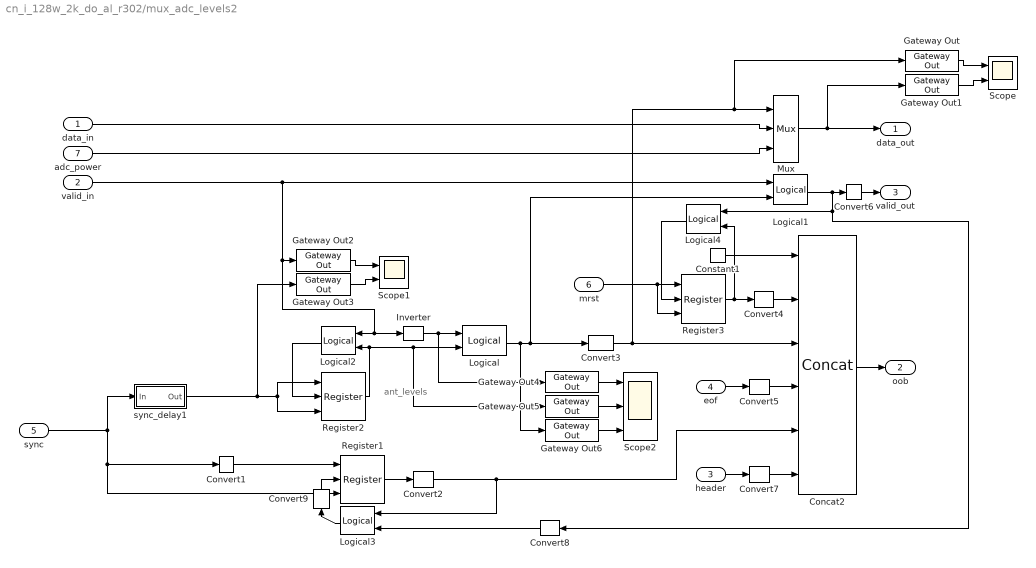
== system cn_i_128w_2k_do_al_r302/mux_adc_levels2 ==
  note: ant_levels
  data_in : Inport  Port=1  LatchInput=off
  valid_in : Inport  Port=2  LatchInput=off
  header : Inport  Port=3  LatchInput=off
  eof : Inport  Port=4  LatchInput=off
  sync : Inport  Port=5  LatchInput=off
  mrst : Inport  Port=6  LatchInput=off
  adc_power : Inport  Port=7  LatchInput=off
  Concat2 : xbsIndex_r3/Concat  num_inputs=6  explicit_period=off  period=1  dbl_ovrd=off
  Constant1 : xbsIndex_r3/Constant  const=0  equ=P=C  arith_type=Unsigned  n_bits=3  bin_pt=0  opselect=C  inp2=PCIN>>17  opr=+  inp1=P  carry=CIN  iostate=0  explicit_period=on  period=1  dbl_ovrd=off
  Convert{1..5,7} (6 alike) : xbsIndex_r3/Convert  arith_type=Unsigned  n_bits=1  bin_pt=0  quantization=Truncate  overflow=Wrap  latency=0  explicit_period=off  period=1  dbl_ovrd=off  show_param=off  inserted_by_tool=off  pipeline=off
      settings: xl_area=[0, 0, 0, 0, 0, 0, 0]
  Convert6 : xbsIndex_r3/Convert  arith_type=Boolean  n_bits=1  bin_pt=0  quantization=Truncate  overflow=Wrap  latency=0  explicit_period=off  period=1  dbl_ovrd=off  show_param=off  inserted_by_tool=off  pipeline=off
      settings: xl_area=[0, 0, 0, 0, 0, 0, 0]
  Convert8 : xbsIndex_r3/Convert  Orientation=left  arith_type=Unsigned  n_bits=1  bin_pt=0  quantization=Truncate  overflow=Wrap  latency=0  explicit_period=off  period=1  dbl_ovrd=off  show_param=off  inserted_by_tool=off  pipeline=off
      settings: xl_area=[0, 0, 0, 0, 0, 0, 0]
  Convert9 : xbsIndex_r3/Convert  Orientation=up  arith_type=Boolean  n_bits=1  bin_pt=0  quantization=Truncate  overflow=Wrap  latency=0  explicit_period=off  period=1  dbl_ovrd=off  show_param=off  inserted_by_tool=off  pipeline=off
      settings: xl_area=[0, 0, 0, 0, 0, 0, 0]
  Gateway Out{,1..6} (7 alike) : xbsIndex_r3/Gateway Out  output_type=Double  nbits=8  bin_pt=6  arith_type=Boolean  quantization=Truncate  overflow=Wrap  hdl_port=on  timing_constraint=None  locs_specified=off  LOCs={}  needs_fixed_name=off  show_param=off
      settings: xl_area=[0, 0, 0, 0, 0, 0, 0]
  Inverter : xbsIndex_r3/Inverter  latency=0  explicit_period=off  period=1  en=off  dbl_ovrd=off  show_param=off
      settings: xl_area=[0, 0, 0, 0, 0, 0, 0]
  Logical : xbsIndex_r3/Logical  logical_function=AND  inputs=2  precision=Full  arith_type=Unsigned  n_bits=8  bin_pt=2  align_bp=off  latency=0  explicit_period=off  period=1  en=off  dbl_ovrd=off  show_param=off
      settings: xl_area=[0, 0, 0, 0, 0, 0, 0]
  Logical1 : xbsIndex_r3/Logical  logical_function=OR  inputs=2  precision=Full  arith_type=Unsigned  n_bits=8  bin_pt=2  align_bp=on  latency=0  explicit_period=on  period=1  en=off  dbl_ovrd=off  show_param=off
      settings: xl_area=[0, 0, 0, 0, 0, 0, 0]
  Logical2 : xbsIndex_r3/Logical  Orientation=left  logical_function=AND  inputs=2  precision=Full  arith_type=Unsigned  n_bits=1  bin_pt=0  align_bp=off  latency=0  explicit_period=on  period=1  en=off  dbl_ovrd=off  show_param=off
      settings: xl_area=[0, 0, 0, 0, 0, 0, 0]
  Logical3 : xbsIndex_r3/Logical  Orientation=left  logical_function=AND  inputs=2  precision=Full  arith_type=Unsigned  n_bits=1  bin_pt=0  align_bp=off  latency=0  explicit_period=on  period=1  en=off  dbl_ovrd=off  show_param=off
      settings: xl_area=[0, 0, 0, 0, 0, 0, 0]
  Logical4 : xbsIndex_r3/Logical  Orientation=left  logical_function=AND  inputs=2  precision=Full  arith_type=Unsigned  n_bits=1  bin_pt=0  align_bp=off  latency=0  explicit_period=on  period=1  en=off  dbl_ovrd=off  show_param=off
      settings: xl_area=[0, 0, 0, 0, 0, 0, 0]
  Mux : xbsIndex_r3/Mux  inputs=2  precision=Full  arith_type="Signed  (2's comp)"  n_bits=8  bin_pt=2  quantization=Truncate  overflow=Wrap  latency=0  explicit_period=on  period=1  en=off  dbl_ovrd=off  show_param=off  mux_type=off  use_rpm=off  gen_core=off
      settings: xl_area=[0, 0, 0, 0, 0, 0, 0]
  Register1 : xbsIndex_r3/Register  init=0  reg_only_valid=off  explicit_period=on  period=1  rst=on  en=on  out_en=off  dbl_ovrd=off  show_param=off
      settings: xl_area=[0, 0, 0, 0, 0, 0, 0]
  Register2 : xbsIndex_r3/Register  init=0  reg_only_valid=off  explicit_period=on  period=1  rst=on  en=on  out_en=off  dbl_ovrd=off  show_param=off
      settings: xl_area=[0, 0, 0, 0, 0, 0, 0]
  Register3 : xbsIndex_r3/Register  init=0  reg_only_valid=off  explicit_period=on  period=1  rst=on  en=on  out_en=off  dbl_ovrd=off  show_param=off
      settings: xl_area=[0, 0, 0, 0, 0, 0, 0]
  Scope : Scope  NumInputPorts=2
      settings: YMin=0~-1e+022  YMax=2~1.7e+023  SaveName=ScopeData3
  Scope1 : Scope  NumInputPorts=2
      settings: YMin=0~-1e+022  YMax=2~1.7e+023  SaveName=ScopeData2
  Scope2 : Scope  NumInputPorts=3
      settings: YMin=-1.67772e+007~0~-5  YMax=4.5e+023~1~5  SaveName=ScopeData11
  sync_delay1 : Subsystem  mask(sync_delay){DelayLen=wait_time}
      mask prompts: DelayLen "Delay Length:"
      mask help: Delay an infrequent boolean pulse by the specified number of clocks.
      mask init:
      | BitWidth = max(2, ceil(log2(DelayLen+1)));
      | UseCounter = 1;
      | if DelayLen == 0,
      | 	UseCounter = 0;
      | end
      mask Help: eval('xlWeb([getenv(''MLIB_ROOT''), ''\casper_library\doc\sync_delay_usage.html''])')
      mask Display: fprintf('Z^-%d', DelayLen)
  data_out : Outport
  oob : Outport  Port=2
  valid_out : Outport  Port=3
  wires:
  Concat2/1 -> oob/1
  sync/1 -> sync_delay1/1(In), Register1/3, Convert1/1
  Mux/1 -> data_out/1, Gateway Out1/1
  data_in/1 -> Mux/2
  adc_power/1 -> Mux/3
  Logical1/1 -> Logical4/1, Convert8/1, Convert6/1
  valid_in/1 -> Logical1/1, Gateway Out2/1, Logical2/1, Inverter/1
  Register2/1 -> Logical2/2, Gateway Out5/1, Logical/2
  sync_delay1/1(Out) -> Register2/1, Register2/3, Gateway Out3/1
  Gateway Out/1 -> Scope/1
  Gateway Out1/1 -> Scope/2
  Constant1/1 -> Concat2/1
  eof/1 -> Convert5/1
  header/1 -> Convert7/1
  Gateway Out2/1 -> Scope1/1
  Gateway Out3/1 -> Scope1/2
  Logical2/1 -> Register2/2
  Gateway Out4/1 -> Scope2/1
  Gateway Out5/1 -> Scope2/2
  Gateway Out6/1 -> Scope2/3
  Logical/1 -> Gateway Out6/1, Convert3/1, Logical1/2
  Convert3/1 -> Concat2/3, Mux/1, Gateway Out/1
  Inverter/1 -> Gateway Out4/1, Logical/1
  Register1/1 -> Convert2/1
  Register3/1 -> Logical4/2, Convert4/1
  mrst/1 -> Register3/1, Register3/3
  Logical3/1 -> Convert9/1
  Logical4/1 -> Register3/2
  Convert6/1 -> valid_out/1
  Convert4/1 -> Concat2/2
  Convert5/1 -> Concat2/4
  Convert7/1 -> Concat2/6
  Convert2/1 -> Concat2/5, Logical3/1
  Convert8/1 -> Logical3/2
  Convert9/1 -> Register1/2
  Convert1/1 -> Register1/1

== system cn_i_128w_2k_do_al_r302/neg_edge_ext ==
  in : Inport  Port=1  LatchInput=off
  Constant5 : xbsIndex_r3/Constant  const=pulse_len  equ=P=C  arith_type=Unsigned  n_bits=bits  bin_pt=0  opselect=C  inp2=PCIN>>17  opr=+  inp1=P  carry=CIN  iostate=0  explicit_period=off  period=1  dbl_ovrd=off
  Counter3 : xbsIndex_r3/Counter  cnt_type=Free Running  n_bits=bits  bin_pt=0  arith_type=Unsigned  start_count=0  cnt_to=1023  cnt_by_val=1  operation=Up  explicit_period=on  period=1  load_pin=off  rst=on  en=on  dbl_ovrd=off  show_param=off  use_rpm=on  gen_core=off
      settings: xl_area=[0, 0, 0, 0, 0, 0, 0]
  Relational5 : xbsIndex_r3/Relational  mode=a!=b  latency=0  explicit_period=off  period=1  en=off  dbl_ovrd=off  show_param=off
      settings: xl_area=[0, 0, 0, 0, 0, 0, 0]
  out : Outport
  wires:
  in/1 -> Counter3/1
  Relational5/1 -> out/1, Counter3/2
  Constant5/1 -> Relational5/2
  Counter3/1 -> Relational5/1

== system cn_i_128w_2k_do_al_r302/one_ant_a_time ==
  din : Inport  Port=1  LatchInput=off
  sync : Inport  Port=2  LatchInput=off
  Concat2 : xbsIndex_r3/Concat  num_inputs=2  explicit_period=off  period=1  dbl_ovrd=off
  Constant2 : xbsIndex_r3/Constant  const=1  equ=P=C  arith_type=Boolean  n_bits=1  bin_pt=0  opselect=C  inp2=PCIN>>17  opr=+  inp1=P  carry=CIN  iostate=0  explicit_period=on  period=1  dbl_ovrd=off
  Slice11 : xbsIndex_r3/Slice  mode=Lower Bit Location + Width  nbits=16  bit1=0  base1=MSB of Input  bit0=16  base0=LSB of Input  boolean_output=off  explicit_period=off  period=1  dbl_ovrd=off
  Slice7 : xbsIndex_r3/Slice  mode=Lower Bit Location + Width  nbits=16  bit1=0  base1=MSB of Input  bit0=0  base0=LSB of Input  boolean_output=off  explicit_period=off  period=1  dbl_ovrd=off
  reorder : reorder_library/reorder  map=[(0:63)*2, (0:63)*2+1]  n_inputs=1  bram_latency=2  map_latency=0
      link override sync_en_delay/Constant: equ=P=C
      link override sync_en_delay/Constant1: equ=P=C
      link override sync_en_delay/Constant2: equ=P=C
      link override sync_en_delay/Constant3: equ=P=C
  square_transposer : reorder_library/square_transposer  n_inputs=1
  dout : Outport
  sync_out : Outport  Port=2
  wires:
  square_transposer/2 -> Concat2/1
  square_transposer/3 -> Concat2/2
  Slice11/1 -> square_transposer/2
  Slice7/1 -> square_transposer/3
  din/1 -> Slice7/1, Slice11/1
  Concat2/1 -> reorder/3
  Constant2/1 -> reorder/2
  square_transposer/1 -> reorder/1
  sync/1 -> square_transposer/1
  reorder/1 -> sync_out/1
  reorder/3 -> dout/1
